simulink model "compare"  (R2022b)
settings: Solver=FixedStepAuto  StartTime=0.0  StopTime=10  FixedStep=0.005  RelTol=1e-3
values from neighbouring files (symbols this model uses):
  K = y(length(y))/1    [approximate.m]
  T = 2*(t2-t1)    [approximate.m]
  tao = 2*t1-t2+tao0    [approximate.m]
undefined symbols (not defined in the file or in its folder): den, num
settings Model: Creator=31883  LastModifiedBy=Xinrui

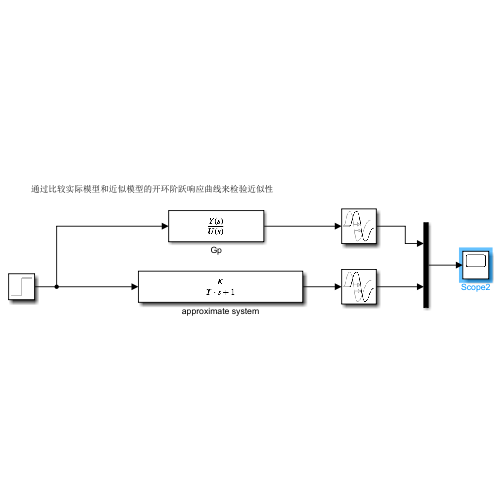
[thumbnail: Simulink's stored preview of the top-level diagram]
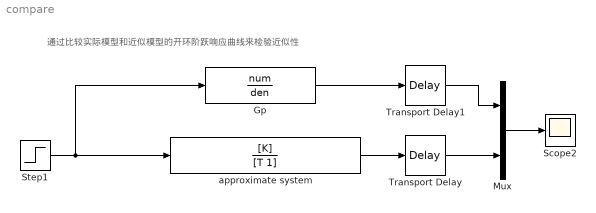
== system compare ==
  note: 通过比较实际模型和近似模型的开环阶跃响应曲线来检验近似性
  Gp : TransferFcn  Numerator=num  Denominator=den
  Mux : Mux  Inputs=2
  Scope2 : Scope
  Step1 : Step  SampleTime=0
  Transport Delay : TransportDelay  DelayTime=tao  BufferSize=2048
  Transport Delay1 : TransportDelay  DelayTime=t  BufferSize=2048
  approximate system : TransferFcn  Numerator=[K]  Denominator=[T 1]
  wires:
  Mux/1 -> Scope2/1
  Step1/1 -> Gp/1, approximate system/1
  approximate system/1 -> Transport Delay/1
  Transport Delay1/1 -> Mux/1
  Transport Delay/1 -> Mux/2
  Gp/1 -> Transport Delay1/1
